simulink model "sampleModel1977"  (R2023a)
settings: Solver=VariableStepAuto  StartTime=0.0  StopTime=10.0  RelTol=1e-3
libraries: hdlsllib x6, simulink x4
settings Model: Creator=user1  LastModifiedBy=user1

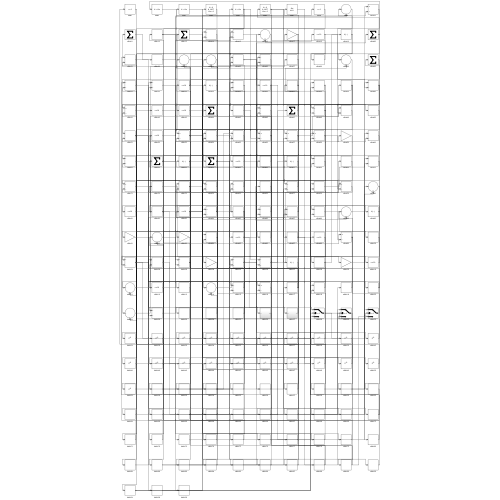
[thumbnail: Simulink's stored preview of the top-level diagram]
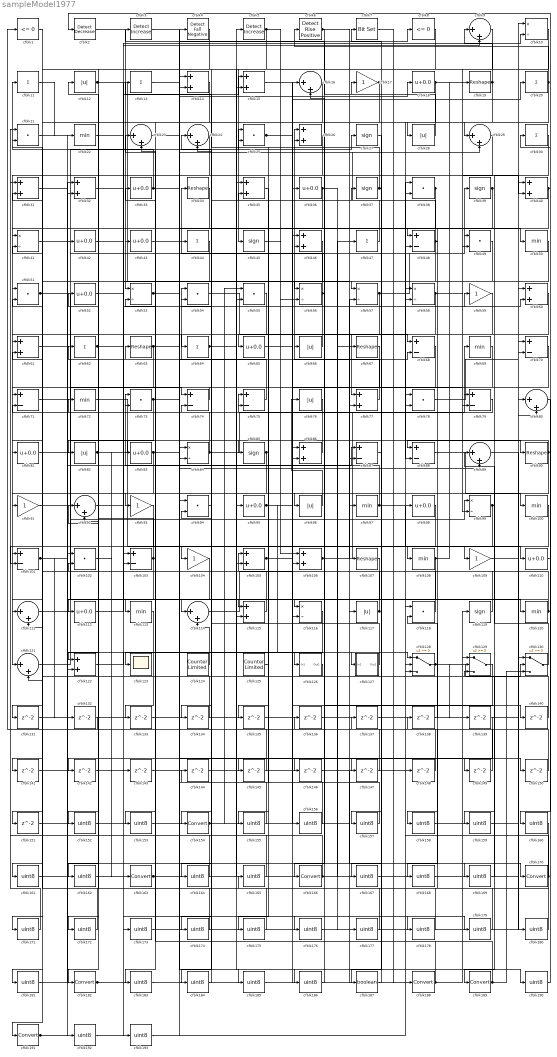
== system sampleModel1977 ==
  cfblk1 : hdlsllib/Logic and Bit Operations/Compare To Zero  relop=<=  OutDataTypeStr=boolean
  cfblk{10,41,53,56..58,84,99,116} (9 alike) : Product  Inputs=*/  RndMeth=Zero  SaturateOnIntegerOverflow=on
  cfblk{22,50,69,72,97,100,108,113,120} (9 alike) : MinMax
  cfblk{48,68,70..71,74..75,79,87..88,101,103} (11 alike) : Sum  Inputs=+-
  cfblk{21,25,38,49,51,54..55,73,78,94,102,118} (12 alike) : DotProduct  OutDataTypeStr=Inherit: Inherit via internal rule
  cfblk{17,59,91,93,104,109} (6 alike) : Gain
  cfblk{14..15,26,31..32,35,40,46,60..61,77,86,105..106,115,122} (16 alike) : Sum
  cfblk{19,34,63,67,90,107} (6 alike) : Reshape
  cfblk{11,13,20,30,44,47,62,64} (8 alike) : Sum  Inputs=+
  cfblk{18,33,36,42..43,52,65,81,83,95,98,110,112} (13 alike) : Bias  Bias=0.0  SaturateOnIntegerOverflow=off
  cfblk{9,16,23..24,29,80,89,92,111,114,121} (11 alike) : Sum  Inputs=|++
  cfblk{12,28,66,76,82,96,117} (7 alike) : Abs  SaturateOnIntegerOverflow=off
  cfblk{27,37,39,45,85,119} (6 alike) : Signum
  cfblk123 : Scope
  cfblk124 : hdlsllib/Sources/Counter Limited  uplimit=7  tsamp=-1
  cfblk125 : hdlsllib/Sources/Counter Limited  uplimit=7  tsamp=-1
  cfblk126 : Subsystem
      settings: LibrarySourceBlock=|
      | hdlsllib/Ports &
      | Subsystems/Subsystem
  cfblk127 : Subsystem
      settings: LibrarySourceBlock=|
      | hdlsllib/Ports &
      | Subsystems/Subsystem
  cfblk128 : Switch  SaturateOnIntegerOverflow=off  InputSameDT=off
  cfblk129 : Switch  SaturateOnIntegerOverflow=off  InputSameDT=off
  cfblk130 : Switch  SaturateOnIntegerOverflow=off  InputSameDT=off
  cfblk{131..151} (21 alike) : Delay  SampleTime=1
  cfblk{152..153,155..162,164..165,167..169,171..181,183..186,190,192..193} (33 alike) : DataTypeConversion  OutDataTypeStr=uint8  SaturateOnIntegerOverflow=off  RndMeth=Floor
  cfblk{154,163,166,170,182,188..189,191} (8 alike) : DataTypeConversion  SaturateOnIntegerOverflow=off  RndMeth=Floor
  cfblk187 : DataTypeConversion  OutDataTypeStr=boolean  SaturateOnIntegerOverflow=off  RndMeth=Floor
  cfblk2 : simulink/Logic and Bit Operations/Detect Decrease  vinit=0.0  OutDataTypeStr=boolean
      settings: LibrarySourceBlock=|
      | hdlsllib/Logic and Bit
      | Operations/Detect
      | Decrease
  cfblk3 : simulink/Logic and Bit Operations/Detect Increase  vinit=0.0  OutDataTypeStr=boolean
      settings: LibrarySourceBlock=|
      | hdlsllib/Logic and Bit
      | Operations/Detect
      | Increase
  cfblk4 : hdlsllib/Logic and Bit Operations/Detect Fall Negative  vinit=0  OutDataTypeStr=boolean
  cfblk5 : simulink/Logic and Bit Operations/Detect Increase  vinit=0.0  OutDataTypeStr=boolean
      settings: LibrarySourceBlock=|
      | hdlsllib/Logic and Bit
      | Operations/Detect
      | Increase
  cfblk6 : hdlsllib/Logic and Bit Operations/Detect Rise Positive  vinit=0  OutDataTypeStr=boolean
  cfblk7 : simulink/Logic and Bit Operations/Bit Set  iBit=0
      settings: LibrarySourceBlock=|
      | hdlsllib/Logic and Bit
      | Operations/Bit Set
  cfblk8 : hdlsllib/Logic and Bit Operations/Compare To Zero  relop=<=  OutDataTypeStr=boolean
  wires:
  cfblk111/1 -> cfblk27/1
  cfblk45/1 -> cfblk106/1
  cfblk95/1 -> cfblk127/1(In1), cfblk20/1
  cfblk103/1 -> cfblk12/1, cfblk112/1
  cfblk25/1 -> cfblk79/2, cfblk140/1
  cfblk126/1(Out1) -> cfblk63/1
  cfblk96/1 -> cfblk76/1
  cfblk34/1 -> cfblk121/1
  cfblk113/1 -> cfblk123/1
  cfblk77/1 -> cfblk26/1
  cfblk61/1 -> cfblk84/2
  cfblk74/1 -> cfblk71/1
  cfblk117/1 -> cfblk105/1, cfblk52/1, cfblk53/2
  cfblk53/1 -> cfblk29/2, cfblk149/1
  cfblk42/1 -> cfblk103/1
  cfblk60/1 -> cfblk106/2
  cfblk58/1 -> cfblk77/1, cfblk60/2
  cfblk2/1 -> cfblk53/1
  cfblk11/1 -> cfblk22/1
  cfblk90/1 -> cfblk88/1, cfblk142/1
  cfblk37/1 -> cfblk13/1, cfblk167/1
  cfblk72/1 -> cfblk110/1
  cfblk121/1 -> cfblk99/1
  cfblk97/1 -> cfblk73/1, cfblk109/1, cfblk148/1
  cfblk114/1 -> cfblk16/1
  cfblk79/1 -> cfblk73/2
  cfblk108/1 -> cfblk19/1, cfblk135/1
  cfblk26/1 -> cfblk51/1
  cfblk66/1 -> cfblk65/1
  cfblk47/1 -> cfblk17/1
  cfblk82/1 -> cfblk90/1, cfblk143/1
  cfblk94/1 -> cfblk154/1
  cfblk5/1 -> cfblk45/1, cfblk56/2, cfblk115/2
  cfblk125/1 -> cfblk75/1
  cfblk119/1 -> cfblk24/1
  cfblk71/1 -> cfblk114/1
  cfblk83/1 -> cfblk18/1, cfblk8/1, cfblk68/2, cfblk161/1
  cfblk98/1 -> cfblk105/2
  cfblk15/1 -> cfblk36/1
  cfblk106/1 -> cfblk69/1, cfblk67/1
  cfblk102/1 -> cfblk163/1
  cfblk30/1 -> cfblk189/1
  cfblk33/1 -> cfblk11/1, cfblk50/1
  cfblk109/1 -> cfblk60/1
  cfblk21/1 -> cfblk42/1
  cfblk12/1 -> cfblk97/1, cfblk56/1
  cfblk115/1 -> cfblk54/1
  cfblk36/1 -> cfblk55/2, cfblk177/1, cfblk183/1
  cfblk81/1 -> cfblk39/1
  cfblk18/1 -> cfblk88/2, cfblk40/2
  cfblk122/1 -> cfblk126/1(In1)
  cfblk49/1 -> cfblk103/2
  cfblk38/1 -> cfblk86/2, cfblk131/1
  cfblk57/1 -> cfblk49/1, cfblk162/1
  cfblk62/1 -> cfblk15/1, cfblk9/2
  cfblk55/1 -> cfblk101/1
  cfblk88/1 -> cfblk100/1
  cfblk54/1 -> cfblk107/1
  cfblk130/1 -> cfblk89/1
  cfblk52/1 -> cfblk25/1
  cfblk105/1 -> cfblk79/1, cfblk147/1
  cfblk31/1 -> cfblk170/1
  cfblk28/1 -> cfblk3/1
  cfblk39/1 -> cfblk48/1, cfblk49/2, cfblk168/1
  cfblk44/1 -> cfblk182/1
  cfblk110/1 -> cfblk2/1
  cfblk124/1 -> cfblk114/2
  cfblk118/1 -> cfblk33/1
  cfblk14/1 -> cfblk191/1
  cfblk87/1 -> cfblk37/1
  cfblk64/1 -> cfblk95/1, cfblk190/1
  cfblk17/1 -> cfblk41/1, cfblk134/1
  cfblk120/1 -> cfblk113/1, cfblk21/2
  cfblk73/1 -> cfblk82/1, cfblk115/1
  cfblk78/1 -> cfblk40/1
  cfblk29/1 -> cfblk104/1
  cfblk19/1 -> cfblk9/1, cfblk28/1, cfblk43/1
  cfblk84/1 -> cfblk58/2, cfblk72/1, cfblk41/2
  cfblk22/1 -> cfblk10/2
  cfblk75/1 -> cfblk54/2
  cfblk9/1 -> cfblk99/2
  cfblk99/1 -> cfblk122/1, cfblk159/1
  cfblk63/1 -> cfblk111/1, cfblk85/1
  cfblk129/1 -> cfblk166/1
  cfblk24/1 -> cfblk93/1
  cfblk51/1 -> cfblk74/1, cfblk120/1
  cfblk128/1 -> cfblk130/2, cfblk139/1
  cfblk127/1(Out1) -> cfblk62/1
  cfblk85/1 -> cfblk91/1, cfblk111/2
  cfblk86/1 -> cfblk35/2
  cfblk76/1 -> cfblk75/2
  cfblk101/1 -> cfblk116/2, cfblk87/1, cfblk132/1
  cfblk16/1 -> cfblk64/1
  cfblk7/1 -> cfblk188/1
  cfblk40/1 -> cfblk108/1, cfblk145/1, cfblk146/1
  cfblk91/1 -> cfblk128/1
  cfblk68/1 -> cfblk81/1
  cfblk3/1 -> cfblk89/2
  cfblk56/1 -> cfblk96/1, cfblk34/1, cfblk181/1
  cfblk48/1 -> cfblk24/2, cfblk57/1, cfblk158/1
  cfblk93/1 -> cfblk101/2
  cfblk1/1 -> cfblk61/1
  cfblk112/1 -> cfblk59/1
  cfblk69/1 -> cfblk121/2
  cfblk20/1 -> cfblk29/1, cfblk6/1
  cfblk104/1 -> cfblk122/2
  cfblk6/1 -> cfblk116/1, cfblk48/2, cfblk68/1
  cfblk131/1 -> cfblk77/2
  cfblk132/1 -> cfblk1/1
  cfblk116/1 -> cfblk133/1
  cfblk133/1 -> cfblk58/1
  cfblk134/1 -> cfblk51/2
  cfblk135/1 -> cfblk10/1
  cfblk136/1 -> cfblk16/2
  cfblk137/1 -> cfblk38/2
  cfblk138/1 -> cfblk118/2
  cfblk140/1 -> cfblk84/1
  cfblk100/1 -> cfblk141/1
  cfblk141/1 -> cfblk86/1
  cfblk144/1 -> cfblk78/1
  cfblk145/1 -> cfblk61/2
  cfblk147/1 -> cfblk35/1
  cfblk148/1 -> cfblk74/2
  cfblk149/1 -> cfblk26/2
  cfblk13/1 -> cfblk150/1
  cfblk150/1 -> cfblk71/2
  cfblk50/1 -> cfblk151/1
  cfblk151/1 -> cfblk15/2
  cfblk4/1 -> cfblk152/1
  cfblk152/1 -> cfblk117/1
  cfblk59/1 -> cfblk153/1
  cfblk153/1 -> cfblk4/1
  cfblk154/1 -> cfblk55/1, cfblk186/1
  cfblk35/1 -> cfblk155/1
  cfblk155/1 -> cfblk94/1
  cfblk65/1 -> cfblk156/1
  cfblk156/1 -> cfblk94/2
  cfblk70/1 -> cfblk157/1
  cfblk157/1 -> cfblk25/2
  cfblk158/1 -> cfblk70/1
  cfblk159/1 -> cfblk70/2
  cfblk80/1 -> cfblk160/1
  cfblk161/1 -> cfblk80/1
  cfblk162/1 -> cfblk80/2
  cfblk163/1 -> cfblk87/2, cfblk5/1
  cfblk8/1 -> cfblk164/1
  cfblk164/1 -> cfblk102/1
  cfblk160/1 -> cfblk165/1
  cfblk165/1 -> cfblk102/2
  cfblk166/1 -> cfblk21/1, cfblk47/1
  cfblk167/1 -> cfblk129/1
  cfblk168/1 -> cfblk129/2
  cfblk146/1 -> cfblk169/1
  cfblk169/1 -> cfblk129/3
  cfblk170/1 -> cfblk128/2, cfblk38/1
  cfblk10/1 -> cfblk171/1
  cfblk171/1 -> cfblk31/1
  cfblk139/1 -> cfblk172/1
  cfblk172/1 -> cfblk31/2
  cfblk92/1 -> cfblk173/1
  cfblk173/1 -> cfblk130/1
  cfblk107/1 -> cfblk174/1
  cfblk174/1 -> cfblk92/1
  cfblk67/1 -> cfblk175/1
  cfblk175/1 -> cfblk92/2
  cfblk23/1 -> cfblk176/1
  cfblk176/1 -> cfblk118/1
  cfblk177/1 -> cfblk23/1
  cfblk143/1 -> cfblk178/1
  cfblk178/1 -> cfblk23/2
  cfblk32/1 -> cfblk179/1
  cfblk179/1 -> cfblk138/1
  cfblk89/1 -> cfblk180/1
  cfblk180/1 -> cfblk32/1
  cfblk181/1 -> cfblk32/2
  cfblk182/1 -> cfblk57/2, cfblk119/1
  cfblk183/1 -> cfblk44/1
  cfblk46/1 -> cfblk184/1
  cfblk184/1 -> cfblk144/1
  cfblk43/1 -> cfblk185/1
  cfblk185/1 -> cfblk46/1
  cfblk186/1 -> cfblk46/2
  cfblk27/1 -> cfblk187/1
  cfblk187/1 -> cfblk7/1
  cfblk188/1 -> cfblk137/1, cfblk136/1
  cfblk189/1 -> cfblk66/1, cfblk130/3, cfblk83/1
  cfblk190/1 -> cfblk30/1
  cfblk191/1 -> cfblk128/3, cfblk98/1, cfblk78/2
  cfblk41/1 -> cfblk192/1
  cfblk192/1 -> cfblk14/1
  cfblk142/1 -> cfblk193/1
  cfblk193/1 -> cfblk14/2

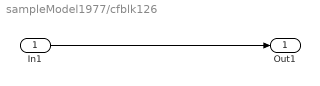
== system sampleModel1977/cfblk126 ==
  In1 : Inport
  Out1 : Outport
  wires:
  In1/1 -> Out1/1

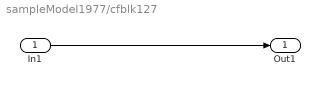
== system sampleModel1977/cfblk127 ==
  In1 : Inport
  Out1 : Outport
  wires:
  In1/1 -> Out1/1
